simulink model "tank_mod_"  (R2020b)
settings: Solver=VariableStepAuto  StartTime=0.0  StopTime=10.0  RelTol=1e-3
values from neighbouring files (symbols this model uses):
  A = [A11 A12 A13 ; A21 A22 A23 ; A31 A32 A33 ]    [codigo_ex.m]    (also in sistema_tanques_control.m; tank_mod.m)
  B = [B11 B12 ; B21 B22 ;B31 B32 ]    [codigo_ex.m]    (also in sistema_tanques_control.m; tank_mod.m)
  K1 = [21.6 3 -5; 2.9 19 -4]*10e-4    [codigo_ex.m]    (also in controlador.m = [0.0216    0.0030   -0.0050; prueba_controlador_cpp.m = [0.0216    0.0030   -0.0050; sistema_tanques_control.m; tank_mod.m)
  K2 = [-0.95 -0.32; -0.3 -0.91]*10e-4    [codigo_ex.m]    (also in controlador.m = 1.0e-03 *K2; prueba_controlador_cpp.m = 1.0e-03 *K2; sistema_tanques_control.m; tank_mod.m)
  tm = 1    [codigo_ex.m]    (also in sistema_tanques_control.m; tank_mod.m)
undefined symbols (not defined in the file or in its folder): C
settings Model: Creator=Acer  LastModifiedBy=Acer

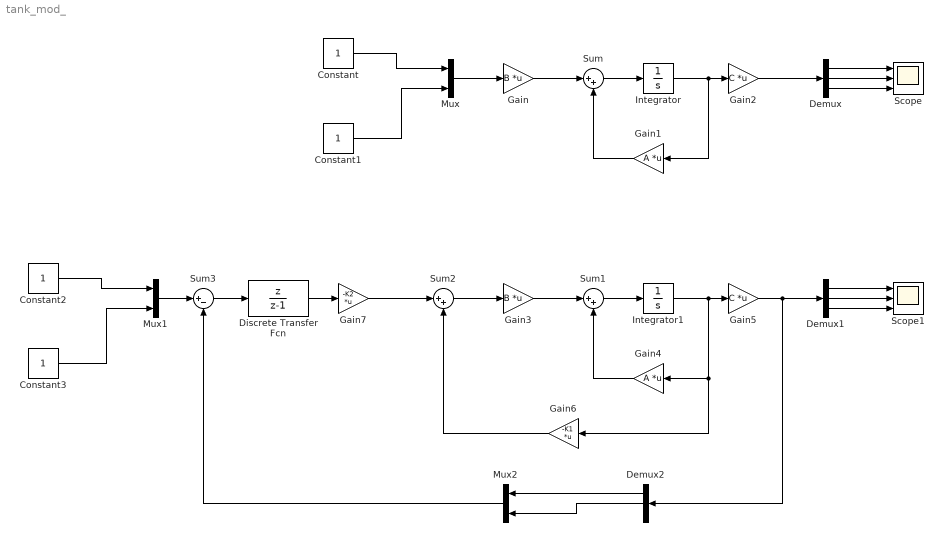
== system tank_mod_ ==
  Constant{,1..3} (4 alike) : Constant
  Demux : Demux  Outputs=3
  Demux1 : Demux  Outputs=3
  Demux2 : Demux  Outputs=3
  Discrete Transfer Fcn : DiscreteTransferFcn  Numerator=[1 0]  Denominator=[1 -1]  SampleTime=tm
  Gain : Gain  Gain=B  Multiplication=Matrix(K*u)
  Gain1 : Gain  Gain=A  Multiplication=Matrix(K*u)
  Gain2 : Gain  Gain=C  Multiplication=Matrix(K*u)
  Gain3 : Gain  Gain=B  Multiplication=Matrix(K*u)
  Gain4 : Gain  Gain=A  Multiplication=Matrix(K*u)
  Gain5 : Gain  Gain=C  Multiplication=Matrix(K*u)
  Gain6 : Gain  Gain=-K1  Multiplication=Matrix(K*u)
  Gain7 : Gain  Gain=-K2  Multiplication=Matrix(K*u)
  Integrator : Integrator
  Integrator1 : Integrator
  Mux : Mux  Inputs=2
  Mux1 : Mux  Inputs=2
  Mux2 : Mux  Inputs=2
  Scope : Scope  NumInputPorts=3
  Scope1 : Scope  NumInputPorts=3
  Sum : Sum  Inputs=|++
  Sum1 : Sum  Inputs=|++
  Sum2 : Sum  Inputs=|++
  Sum3 : Sum  Inputs=|+-
  wires:
  Constant/1 -> Mux/1
  Constant1/1 -> Mux/2
  Mux/1 -> Gain/1
  Gain2/1 -> Demux/1
  Gain/1 -> Sum/1
  Sum/1 -> Integrator/1
  Gain1/1 -> Sum/2
  Integrator/1 -> Gain2/1, Gain1/1
  Demux/1 -> Scope/1
  Demux/2 -> Scope/2
  Demux/3 -> Scope/3
  Demux1/1 -> Scope1/1
  Gain5/1 -> Demux2/1, Demux1/1
  Gain4/1 -> Sum1/2
  Sum1/1 -> Integrator1/1
  Gain3/1 -> Sum1/1
  Integrator1/1 -> Gain5/1, Gain6/1, Gain4/1
  Demux1/3 -> Scope1/3
  Demux1/2 -> Scope1/2
  Sum2/1 -> Gain3/1
  Gain6/1 -> Sum2/2
  Gain7/1 -> Sum2/1
  Constant2/1 -> Mux1/1
  Constant3/1 -> Mux1/2
  Mux1/1 -> Sum3/1
  Demux2/1 -> Mux2/1
  Demux2/2 -> Mux2/2
  Mux2/1 -> Sum3/2
  Sum3/1 -> Discrete Transfer Fcn/1
  Discrete Transfer Fcn/1 -> Gain7/1
